simulink model "BrowarModel"  (R2024a)
settings: Solver=ode5  StartTime=0.0  StopTime=inf  FixedStep=0.1  RelTol=1e-3
undefined symbols (not defined in the file or in its folder): localhost, Matrikon, OI
libraries: opclib x24
(part 8 of 9)

== system BrowarModel/Kadz filtracji/Kadz filtracji/Zbiornik gorny/Silnik elektryczny ==
  note: Silnik elektryczny
  note: Uszkodzenie silnika
  Zalaczenie : Inport
  Zadane obroty : Inport  Port=2
  Obciazenie zew : Inport  Port=3
  Uszkodzenie : Inport  Port=4
  Abs : Abs  SaturateOnIntegerOverflow=off
  Add : Sum
  Add1 : Sum  Inputs=+-
  Const : Constant
  Gain : Gain
  "Hz -> obr/min" : Gain  Gain=60/2
  Inercja mechaniczna : TransferFcn  Denominator=[1 1]
  Poslizg : DotProduct  OutDataTypeStr=Inherit: Inherit via internal rule
  Poslizg jalowy : Constant  Value=0.04
  Poslizg od obciazenia : Gain  Gain=0.05
  Prad jalowy : Gain  Gain=0.5
  Prad nominalny (10A) : Constant  Value=10
  Relay : Relay  OnOutputValue=0  OffOutputValue=1
  Saturation [0,1] : Saturate  UpperLimit=1  LowerLimit=0
  "Saturation [0,1] " : Saturate  UpperLimit=1  LowerLimit=0
  Stan : Subsystem
  Sterowanie : Subsystem
  Sterownik : Subsystem
  Sum : Sum  Inputs=|+-
  Sum1 : Sum  Inputs=|++
  Sum2 : Sum  Inputs=|+-
  Sum3 : Sum  Inputs=|++
  Wplyw uszkodzenia : DotProduct  OutDataTypeStr=Inherit: Inherit via internal rule
  Wplyw obciazenia : DotProduct  OutDataTypeStr=Inherit: Inherit via internal rule
  Wplyw obrotow : DotProduct  OutDataTypeStr=Inherit: Inherit via internal rule
  Zaklocenia : Subsystem
  Zalaczony : DotProduct  OutDataTypeStr=Inherit: Inherit via internal rule
  "obr/min -> FS  " : Gain  Gain=1/1500
  "obr/min -> Hz" : Gain  Gain=1/60*2
  Obroty : Outport
  Prad : Outport  Port=2
  Idle : Outport  Port=3
  Running : Outport  Port=4
  Alarm : Outport  Port=5
  wires:
  Inercja mechaniczna/1 -> Obroty/1, Poslizg/1, Add1/2, "obr/min -> Hz"/1
  Sum/1 -> Inercja mechaniczna/1
  "Hz -> obr/min"/1 -> Sum2/1, Zaklocenia/1(In)  "[obr/min]"
  Poslizg/1 -> Sum/2
  Sum3/1 -> Poslizg/2
  Poslizg od obciazenia/1 -> Sum3/1
  Obciazenie zew/1 -> Saturation [0,1]/1  "FS"
  Poslizg jalowy/1 -> Sum3/2
  Prad nominalny (10A)/1 -> Prad jalowy/1  "A"
  Prad jalowy/1 -> Sum1/2, Wplyw obciazenia/2
  Wplyw obciazenia/1 -> Sum1/1
  Abs/1 -> Wplyw obciazenia/1  "FS"
  Const/1 -> Wplyw obrotow/1
  "obr/min -> Hz"/1 -> Sterownik/1(PV)
  Saturation [0,1]/1 -> Add/2
  Add/1 -> Poslizg od obciazenia/1, Abs/1  "FS"
  Add1/1 -> "obr/min -> FS  "/1
  "obr/min -> FS  "/1 -> Gain/1
  "Saturation [0,1] "/1 -> Add/1
  Zalaczenie/1 -> Sterowanie/2(Zalaczenie), Stan/1(Zalaczony)
  Sterowanie/1(Sterowanie) -> Sterownik/2(SP)
  Gain/1 -> "Saturation [0,1] "/1
  Uszkodzenie/1 -> Relay/1
  Sterownik/1(CV) -> Wplyw uszkodzenia/1
  Relay/1 -> Wplyw uszkodzenia/2, Stan/2(Zdatny)
  Wplyw uszkodzenia/1 -> "Hz -> obr/min"/1
  Wplyw obrotow/1 -> Prad/1  "A"
  Sum1/1 -> Zalaczony/1  "A"
  Zalaczony/1 -> Wplyw obrotow/2
  Zadane obroty/1 -> Sterowanie/1(Zadane obroty)
  Stan/1(Idle) -> Idle/1
  Stan/2(Running) -> Running/1, Zalaczony/2
  Stan/3(Alarm) -> Alarm/1
  Sum2/1 -> Add1/1, Sum/1
  Zaklocenia/1(Out) -> Sum2/2

== system BrowarModel/Kadz warzelna/Kadz warzelna/Model akumulacji ciepla w zbiorniku z ciecza/Cieplo strumienia cieczy doplywajacej ==
  Temperatura strumienia cieczy : Inport
  Strumien cieczy : Inport  Port=2
  "  Dot " : DotProduct  OutDataTypeStr=Inherit: Inherit via internal rule
  Cieplo wlasciwe : Constant  Value=4189.9
  Dot : DotProduct  OutDataTypeStr=Inherit: Inherit via internal rule
  Gestosc cieczy : Gain  Gain=1000
  Sum9 : Sum  Inputs=|++
  "Zamiana C->K " : Constant  Value=273.6
  Strumien ciepla : Outport
  wires:
  Cieplo wlasciwe/1 -> Dot/1  "J/(kg*K)"
  Sum9/1 -> Dot/2  "dec K"
  "Zamiana C->K "/1 -> Sum9/2
  Dot/1 -> "  Dot "/1
  Gestosc cieczy/1 -> "  Dot "/2  "kg/s"
  Temperatura strumienia cieczy/1 -> Sum9/1
  "  Dot "/1 -> Strumien ciepla/1  "J/s"
  Strumien cieczy/1 -> Gestosc cieczy/1

== system BrowarModel/Kadz warzelna/Kadz warzelna/Model akumulacji ciepla w zbiorniku z ciecza/Cieplo strumienia cieczy odplywajacej ==
  Temperatura strumienia cieczy : Inport
  Strumien cieczy : Inport  Port=2
  " Dot " : DotProduct  OutDataTypeStr=Inherit: Inherit via internal rule
  Cieplo wlasciwe : Constant  Value=4189.9
  "Dot " : DotProduct  OutDataTypeStr=Inherit: Inherit via internal rule
  Gestosc : Gain  Gain=1000
  Strumien ciepla : Outport
  wires:
  "Dot "/1 -> " Dot "/2
  Cieplo wlasciwe/1 -> "Dot "/2  "J/(kg*K)"
  Temperatura strumienia cieczy/1 -> " Dot "/1  "decK"
  Strumien cieczy/1 -> Gestosc/1  "m3/s"
  " Dot "/1 -> Strumien ciepla/1  "J/s"
  Gestosc/1 -> "Dot "/1  "kg/s"

== system BrowarModel/Kadz warzelna/Kadz warzelna/Model jakosci warzenia/Gotowanie  ==
  Srednia temperatura : Inport
  Jakosc mieszaniny : Inport  Port=2
  Objetosc mieszaniny : Inport  Port=3
  Odplyw : Inport  Port=4
  Booster : Product  RndMeth=Zero
  Booster block : Subsystem
  Display : Display
  Display1 : Display
  Divide : Product  Inputs=*/
  Dynamika rozkladu : Gain  Gain=1/1000
  Ilosc : Integrator  LimitOutput=on  UpperSaturationLimit=48  LowerSaturationLimit=0
  Nasycenie : DotProduct  OutDataTypeStr=Inherit: Inherit via internal rule
  "Odplyw " : DotProduct  OutDataTypeStr=Inherit: Inherit via internal rule
  Relational Operator1 : RelationalOperator  Operator=>  InputSameDT=off
  Sum8 : Sum  Inputs=|+-
  Sum9 : Sum  Inputs=|+-
  Szybkosc reakcji : DotProduct  OutDataTypeStr=Inherit: Inherit via internal rule
  Warunki rozkladu : DotProduct  OutDataTypeStr=Inherit: Inherit via internal rule
  Wplyw temperatury : Lookup  InputValues=[0, 80, 90, 95, 100]  Table=[0, 0, 0.9, 1, 1]  SaturateOnIntegerOverflow=off
  Jakosc : Outport
  wires:
  Wplyw temperatury/1 -> Warunki rozkladu/2, Display/1
  Warunki rozkladu/1 -> Dynamika rozkladu/1
  Ilosc/1 -> Sum8/2, Divide/1
  Divide/1 -> "Odplyw "/2, Relational Operator1/2, Jakosc/1, Display1/1
  Relational Operator1/1 -> Nasycenie/1
  Sum8/1 -> Szybkosc reakcji/2
  Sum9/1 -> Ilosc/1
  Nasycenie/1 -> Sum9/1
  "Odplyw "/1 -> Sum9/2
  Srednia temperatura/1 -> Wplyw temperatury/1
  Objetosc mieszaniny/1 -> Divide/2, Sum8/1
  Odplyw/1 -> "Odplyw "/1
  Jakosc mieszaniny/1 -> Warunki rozkladu/1, Relational Operator1/1
  Booster block/1(Out) -> Booster/1
  Szybkosc reakcji/1 -> Nasycenie/2
  Dynamika rozkladu/1 -> Booster/2
  Booster/1 -> Szybkosc reakcji/1

== system BrowarModel/Kadz warzelna/Kadz warzelna/Model ogrzewacza/Booster  ==
  In1 : Inport
  In2 : Inport  Port=2
  Switch : Switch  Threshold=0.5  SaturateOnIntegerOverflow=off  InputSameDT=off
  Out : Outport
  wires:
  [TrybSym] -> Switch/2
  In1/1 -> Switch/1
  Switch/1 -> Out/1
  In2/1 -> Switch/3

== system BrowarModel/Kadz warzelna/Kadz warzelna/Model ogrzewacza/Booster block ==
  Fast : Constant  Value=2
  Normal : Constant
  Switch : Switch  Threshold=0.5  SaturateOnIntegerOverflow=off  InputSameDT=off
  Out : Outport
  wires:
  [TrybSym] -> Switch/2
  Fast/1 -> Switch/1
  Normal/1 -> Switch/3
  Switch/1 -> Out/1

== system BrowarModel/Kadz warzelna/Kadz warzelna/Model ogrzewacza/Zaklocenia ==
  note: Zaklocenia procesowe
  In : Inport
  Product3 : Product  InputSameDT=on  RndMeth=Zero  SaturateOnIntegerOverflow=on  OutDataTypeStr=Inherit: Same as first input
  Product4 : Product  InputSameDT=on  RndMeth=Zero  SaturateOnIntegerOverflow=on  OutDataTypeStr=Inherit: Same as first input
  Random Number : RandomNumber  Seed=4365624  SampleTime=0.1
  Transfer Fcn1 : TransferFcn  Denominator=[10 1]
  Transfer Fcn2 : TransferFcn  Denominator=[10 1]
  Transfer Fcn3 : TransferFcn  Denominator=[10 1]
  Out : Outport
  wires:
  [ZaklProc] -> Product3/2
  Random Number/1 -> Product3/1
  Product3/1 -> Transfer Fcn1/1
  Transfer Fcn1/1 -> Transfer Fcn2/1
  In/1 -> Product4/1
  Product4/1 -> Out/1
  Transfer Fcn2/1 -> Transfer Fcn3/1
  Transfer Fcn3/1 -> Product4/2

== system BrowarModel/Kadz warzelna/Kadz warzelna/Model rozkladu temperatur/Model rozkladu temperatur ==
  Poziom : Inport
  Temperatura otoczenia : Inport  Port=2
  Srednia temperatura : Inport  Port=3
  "  1/2  " : Gain  Gain=0.5
  "  1/2  1" : Gain  Gain=2
  " Dot  1" : DotProduct  OutDataTypeStr=Inherit: Inherit via internal rule
  "1/2  " : Gain  Gain=0.5
  Max gradient : Gain  Gain=0.9
  MinMax : MinMax
  Mux : Mux  Inputs=2
  Poziom FS : Gain  Gain=1/3
  Sat doplyw Sat FS1 : Saturate  UpperLimit=1  LowerLimit=0
  Saturation : Saturate  UpperLimit=100  LowerLimit=0
  Saturation1 : Saturate  UpperLimit=100  LowerLimit=0
  Saturation2 : Saturate  UpperLimit=100  LowerLimit=0
  Sum1 : Sum  Inputs=|++
  Sum2 : Sum  Inputs=|-+
  Sum3 : Sum  Inputs=|+-
  Sum4 : Sum  Inputs=|-+
  Sum5 : Sum  Inputs=|++
  Sum7 : Sum  Inputs=|-+
  Sum8 : Sum  Inputs=|++
  Transfer Fcn : TransferFcn  Denominator=[10 1]
  Temperatura przy powierzchni : Outport
  Temperatura przy dnie : Outport  Port=2
  Gradient temperatury : Outport  Port=3
  wires:
  Srednia temperatura/1 -> Sum8/2, Sum4/2, Sum1/2, Sum2/2, Sum3/2, Sum5/2, Sum7/2
  Transfer Fcn/1 -> Sat doplyw Sat FS1/1
  Max gradient/1 -> Transfer Fcn/1
  Poziom FS/1 -> Max gradient/1
  Sat doplyw Sat FS1/1 -> " Dot  1"/1
  Sum4/1 -> " Dot  1"/2
  " Dot  1"/1 -> "1/2  "/1, "  1/2  "/1
  "1/2  "/1 -> Sum1/1
  "  1/2  "/1 -> Sum2/1
  Sum2/1 -> Saturation/1
  Sum1/1 -> Saturation1/1
  Saturation1/1 -> Sum3/1
  Saturation/1 -> Sum5/1
  Sum5/1 -> Mux/1
  Sum3/1 -> Mux/2
  Mux/1 -> MinMax/1
  MinMax/1 -> Saturation2/1
  Saturation2/1 -> Sum8/1, Sum7/1, "  1/2  1"/1
  Poziom/1 -> Poziom FS/1
  Temperatura otoczenia/1 -> Sum4/1
  Sum7/1 -> Temperatura przy powierzchni/1
  "  1/2  1"/1 -> Gradient temperatury/1
  Sum8/1 -> Temperatura przy dnie/1

== system BrowarModel/Kadz warzelna/Kadz warzelna/Odplyw z kadzi/Silnik elektryczny ==
  note: Silnik elektryczny
  note: Uszkodzenie silnika
  Zalaczenie : Inport
  Zadane obroty : Inport  Port=2
  Obciazenie zew : Inport  Port=3
  Uszkodzenie : Inport  Port=4
  Abs : Abs  SaturateOnIntegerOverflow=off
  Add : Sum
  Add1 : Sum  Inputs=+-
  Const : Constant
  Gain : Gain
  "Hz -> obr/min" : Gain  Gain=60/2
  Inercja mechaniczna : TransferFcn  Denominator=[1 1]
  Poslizg : DotProduct  OutDataTypeStr=Inherit: Inherit via internal rule
  Poslizg jalowy : Constant  Value=0.04
  Poslizg od obciazenia : Gain  Gain=0.05
  Prad jalowy : Gain  Gain=0.5
  Prad nominalny (10A) : Constant  Value=10
  Relay : Relay  OnOutputValue=0  OffOutputValue=1
  Saturation [0,1] : Saturate  UpperLimit=1  LowerLimit=0
  "Saturation [0,1] " : Saturate  UpperLimit=1  LowerLimit=0
  Stan : Subsystem
  Sterowanie : Subsystem
  Sterownik : Subsystem
  Sum : Sum  Inputs=|+-
  Sum1 : Sum  Inputs=|++
  Sum2 : Sum  Inputs=|+-
  Sum3 : Sum  Inputs=|++
  Wplyw uszkodzenia : DotProduct  OutDataTypeStr=Inherit: Inherit via internal rule
  Wplyw obciazenia : DotProduct  OutDataTypeStr=Inherit: Inherit via internal rule
  Wplyw obrotow : DotProduct  OutDataTypeStr=Inherit: Inherit via internal rule
  Zaklocenia : Subsystem
  Zalaczony : DotProduct  OutDataTypeStr=Inherit: Inherit via internal rule
  "obr/min -> FS  " : Gain  Gain=1/1500
  "obr/min -> Hz" : Gain  Gain=1/60*2
  Obroty : Outport
  Prad : Outport  Port=2
  Idle : Outport  Port=3
  Running : Outport  Port=4
  Alarm : Outport  Port=5
  wires:
  Inercja mechaniczna/1 -> Obroty/1, Poslizg/1, Add1/2, "obr/min -> Hz"/1
  Sum/1 -> Inercja mechaniczna/1
  "Hz -> obr/min"/1 -> Sum2/1, Zaklocenia/1(In)  "[obr/min]"
  Poslizg/1 -> Sum/2
  Sum3/1 -> Poslizg/2
  Poslizg od obciazenia/1 -> Sum3/1
  Obciazenie zew/1 -> Saturation [0,1]/1  "FS"
  Poslizg jalowy/1 -> Sum3/2
  Prad nominalny (10A)/1 -> Prad jalowy/1  "A"
  Prad jalowy/1 -> Sum1/2, Wplyw obciazenia/2
  Wplyw obciazenia/1 -> Sum1/1
  Abs/1 -> Wplyw obciazenia/1  "FS"
  Const/1 -> Wplyw obrotow/1
  "obr/min -> Hz"/1 -> Sterownik/1(PV)
  Saturation [0,1]/1 -> Add/2
  Add/1 -> Poslizg od obciazenia/1, Abs/1  "FS"
  Add1/1 -> "obr/min -> FS  "/1
  "obr/min -> FS  "/1 -> Gain/1
  "Saturation [0,1] "/1 -> Add/1
  Zalaczenie/1 -> Sterowanie/2(Zalaczenie), Stan/1(Zalaczony)
  Sterowanie/1(Sterowanie) -> Sterownik/2(SP)
  Gain/1 -> "Saturation [0,1] "/1
  Uszkodzenie/1 -> Relay/1
  Sterownik/1(CV) -> Wplyw uszkodzenia/1
  Relay/1 -> Wplyw uszkodzenia/2, Stan/2(Zdatny)
  Wplyw uszkodzenia/1 -> "Hz -> obr/min"/1
  Wplyw obrotow/1 -> Prad/1  "A"
  Sum1/1 -> Zalaczony/1  "A"
  Zalaczony/1 -> Wplyw obrotow/2
  Zadane obroty/1 -> Sterowanie/1(Zadane obroty)
  Stan/1(Idle) -> Idle/1
  Stan/2(Running) -> Running/1, Zalaczony/2
  Stan/3(Alarm) -> Alarm/1
  Sum2/1 -> Add1/1, Sum/1
  Zaklocenia/1(Out) -> Sum2/2

== system BrowarModel/Kadz warzelna/Kadz warzelna/Odplyw z kadzi/Zawor dyskretny ==
  note: Model zaworu dyskretnego
  Sterowanie : Inport
  Cisnienie : Inport  Port=2
  Przeciek : Inport  Port=3
  Dlawienie : Inport  Port=4
  Const : Constant  Value=100
  GUIMon : Gain
  Gain : Gain  Gain=(0.15/sqrt(300))/100
  Gain1 : Gain  Gain=1/100
  Integer Delay : Delay  DelayLength=15
  Math Function : Math  Operator=sqrt  SignedPower=on
  Product : Product  RndMeth=Zero
  Product1 : Product  RndMeth=Zero
  Relay : Relay  OnOutputValue=100
  Sat (0-100) : Saturate  UpperLimit=100  LowerLimit=0
  Sat dlawienia (0-100) : Saturate  UpperLimit=100  LowerLimit=0
  Sat przecieku (0-100) : Saturate  UpperLimit=100  LowerLimit=0
  Sum3 : Sum  Inputs=|+-
  Sum4 : Sum  Inputs=|++
  Transfer Fcn : TransferFcn  Denominator=[0.2 1]
  Przeplyw : Outport
  wires:
  Const/1 -> Sum3/1
  Sat dlawienia (0-100)/1 -> Sum3/2
  Sum3/1 -> Gain1/1
  Sat (0-100)/1 -> Product/1
  Sum4/1 -> Sat (0-100)/1
  Relay/1 -> GUIMon/1
  Sat przecieku (0-100)/1 -> Sum4/2
  Sterowanie/1 -> Relay/1
  Product/1 -> Product1/2  "[0,1]"
  Przeciek/1 -> Sat przecieku (0-100)/1
  Dlawienie/1 -> Sat dlawienia (0-100)/1
  Product1/1 -> Transfer Fcn/1
  Gain/1 -> Integer Delay/1  "m3/s"
  Cisnienie/1 -> Math Function/1  "kPa"
  Math Function/1 -> Product1/1
  Transfer Fcn/1 -> Gain/1
  Integer Delay/1 -> Przeplyw/1
  GUIMon/1 -> Sum4/1
  Gain1/1 -> Product/2

== system BrowarModel/Kadz zacierna/Kadz zacierna/Kadz zacierna/Model akumulacji ciepla w zbiorniku z ciecza ==
  note: Model akumulacji ciepla w zbiorniku
  Objetosc cieczy w zbiorniku : Inport
  Przepelnienie : Inport  Port=2
  Strumien odplywu cieczy : Inport  Port=3
  Strumien doplywu wody : Inport  Port=4
  Strumien sruty : Inport  Port=5
  Temperatura strumien doplywu wody : Inport  Port=6
  Temperatura strumien doplywu sruty : Inport  Port=7
  Strumien cieplna dostepny : Inport  Port=8
  Strumien cieplo traconego : Inport  Port=9
  1/gestosc cieczy : Gain  Gain=1/1000
  Cieplo : Integrator  InitialCondition=1238534.44  LimitOutput=on  LowerSaturationLimit=0
  Cieplo parowania : Constant  Value=2257000
  Cieplo strumienia cieczy odplywajacej : Subsystem
  Cieplo strumienia doplywajacego : Subsystem
  "Cieplo wlasciwe " : Constant  Value=4189.9
  Divide : Product  Inputs=/*
  Divide1 : Product  Inputs=*/
  Divide2 : Product  Inputs=*/
  "Dot " : DotProduct  OutDataTypeStr=Inherit: Inherit via internal rule
  Dot 1 : DotProduct  OutDataTypeStr=Inherit: Inherit via internal rule
  Gestosc cieczy : Gain  Gain=1000
  Saturation : Saturate  UpperLimit=inf  LowerLimit=0
  Sum{1..2,4..5} (4 alike) : Sum  Inputs=|+-
  Sum10 : Sum  Inputs=|++
  Sum3 : Sum  Inputs=|-+
  Sum7 : Sum  Inputs=|++
  Switch : Switch  Threshold=0.5  SaturateOnIntegerOverflow=off  InputSameDT=off
  Switch1 : Switch  Threshold=-0.5  SaturateOnIntegerOverflow=off  InputSameDT=off
  Temperatura parowania : Constant  Value=100
  Zamiana C->K : Constant  Value=273.6
  Zero : Constant  Value=0
  Srumien cieczy odparowanej : Outport
  Srednia temperaturacie czy : Outport  Port=2
  wires:
  Strumien odplywu cieczy/1 -> Sum7/1  "m3/s"
  Sum7/1 -> Cieplo strumienia cieczy odplywajacej/2(Strumien cieczy)
  Gestosc cieczy/1 -> Divide/1, "Dot "/2  "kg"
  Objetosc cieczy w zbiorniku/1 -> Gestosc cieczy/1  "m3"
  Cieplo parowania/1 -> Divide2/2  "J/kg"
  Divide2/1 -> 1/gestosc cieczy/1  "kg/s"
  1/gestosc cieczy/1 -> Srumien cieczy odparowanej/1, Sum7/2  "m3/s"
  Sum2/1 -> Cieplo/1  "J/s"
  "Dot "/1 -> Sum2/2, Divide2/1  "J/s"
  Dot 1/1 -> "Dot "/1
  Saturation/1 -> Dot 1/1
  Sum4/1 -> Saturation/1
  Temperatura parowania/1 -> Sum4/2  "dec C"
  Sum10/1 -> Sum2/1  "J/s"
  Sum1/1 -> Sum10/1  "J/s"
  Strumien cieplo traconego/1 -> Sum1/2  "J/s"
  Sum3/1 -> Sum1/1  "J/s"
  Cieplo/1 -> Divide/2  "J"
  Divide/1 -> Divide1/1
  Divide1/1 -> Cieplo strumienia cieczy odplywajacej/1(Temperatura strumienia cieczy), Sum5/1  "dec K"
  Temperatura strumien doplywu wody/1 -> Cieplo strumienia doplywajacego/1(Temperatura strumienia wody)  "dec C"
  "Cieplo wlasciwe "/1 -> Dot 1/2, Divide1/2  "J/(kg*K)"
  Zamiana C->K/1 -> Sum5/2
  Strumien doplywu wody/1 -> Cieplo strumienia doplywajacego/2(Strumien wody)  "m3/s"
  Sum5/1 -> Sum4/1, Srednia temperaturacie czy/1
  Strumien cieplna dostepny/1 -> Sum10/2  "J/s"
  Strumien sruty/1 -> Cieplo strumienia doplywajacego/4(Strumien sruty)
  Temperatura strumien doplywu sruty/1 -> Cieplo strumienia doplywajacego/3(Temperatura strumienia sruty)
  Przepelnienie/1 -> Switch/2, Switch1/2
  Cieplo strumienia doplywajacego/1(Strumien ciepla) -> Switch/3  "J/s"
  Switch/1 -> Sum3/2
  Cieplo strumienia cieczy odplywajacej/1(Strumien ciepla) -> Switch/1, Switch1/1  "J/s"
  Switch1/1 -> Sum3/1
  Zero/1 -> Switch1/3

== system BrowarModel/Kadz zacierna/Kadz zacierna/Kadz zacierna/Model jakosci zacieru ==
  note: Model jakosci zacieru
  Srednia temperatura : Inport
  Odplyw : Inport  Port=2
  Doplyw wody : Inport  Port=3
  Doplyw srutu : Inport  Port=4
  Obroty mieszadla : Inport  Port=5
  Constant : Constant  Value=48
  Display{,1..3} (4 alike) : Display
  Divide : Product  Inputs=*/
  Divide1 : Product  Inputs=/*
  Jakosc mieszaniny : Lookup  InputValues=[0, 0.5 0.75, 1]  Table=[0, 0.1 1, 0]  SaturateOnIntegerOverflow=off
  Objetosc srutu : Integrator  InitialCondition=0.001  LimitOutput=on  UpperSaturationLimit=48  LowerSaturationLimit=0.001
  Objetosc wody : Integrator  InitialCondition=0.001  LimitOutput=on  UpperSaturationLimit=48  LowerSaturationLimit=0.001
  Obroty skalowanie : Gain  Gain=1/2
  Odplyw srutu : DotProduct  OutDataTypeStr=Inherit: Inherit via internal rule
  Odplyw wody : DotProduct  OutDataTypeStr=Inherit: Inherit via internal rule
  Przepelnienie - srut : DotProduct  OutDataTypeStr=Inherit: Inherit via internal rule
  Przepelnienie - woda : DotProduct  OutDataTypeStr=Inherit: Inherit via internal rule
  "Przerwa bialkowa " : Subsystem
  Przerwa dekstrynujaca : Subsystem
  Przerwa maltozowa : Subsystem
  Relational Operator : RelationalOperator  Operator=<  InputSameDT=off
  Sat doplyw Sat FS : Saturate  UpperLimit=1  LowerLimit=0
  Saturation : Saturate  UpperLimit=inf  LowerLimit=0
  Sum5 : Sum  Inputs=-+
  Sum6 : Sum  Inputs=+-
  Sum7 : Sum
  Jakosc : Outport
  wires:
  Sum6/1 -> Objetosc srutu/1
  Odplyw srutu/1 -> Sum6/2
  Objetosc wody/1 -> Sum7/1, Divide/1
  Objetosc srutu/1 -> Sum7/2, Divide1/2
  Sum7/1 -> Divide1/1, Divide/2, Relational Operator/1, "Przerwa bialkowa "/3(Objetosc mieszaniny), Przerwa maltozowa/4(Objetosc mieszaniny), Przerwa dekstrynujaca/4(Objetosc mieszaniny)  "m3"
  Odplyw wody/1 -> Sum5/1
  Divide/1 -> Odplyw wody/1, Jakosc mieszaniny/1
  Divide1/1 -> Odplyw srutu/2
  Sum5/1 -> Objetosc wody/1
  Przepelnienie - woda/1 -> Sum5/2
  Przepelnienie - srut/1 -> Sum6/1
  Relational Operator/1 -> Przepelnienie - woda/2, Przepelnienie - srut/1
  Constant/1 -> Relational Operator/2
  "Przerwa bialkowa "/1(Skrobia rozpuszczona) -> Przerwa maltozowa/1(Skrobia rozpuszczona), Display1/1
  Przerwa maltozowa/1(Dekstryny) -> Przerwa dekstrynujaca/1(Dekstryny), Display2/1
  Srednia temperatura/1 -> "Przerwa bialkowa "/1(Srednia temperatura), Przerwa maltozowa/2(Srednia temperatura), Przerwa dekstrynujaca/2(Srednia temperatura)  "decC"
  Odplyw/1 -> Odplyw wody/2, Odplyw srutu/1, Przerwa dekstrynujaca/5(Odplyw), "Przerwa bialkowa "/4(Odplyw), Przerwa maltozowa/5(Odplyw)  "m3/s"
  Doplyw wody/1 -> Przepelnienie - woda/1  "m3/s"
  Doplyw srutu/1 -> Przepelnienie - srut/2  "m3/s"
  Przerwa dekstrynujaca/1(Maltoza) -> Saturation/1, Display3/1
  Jakosc mieszaniny/1 -> "Przerwa bialkowa "/2(Jakosc mieszaniny), Przerwa maltozowa/3(Jakosc mieszaniny), Przerwa dekstrynujaca/3(Jakosc mieszaniny), Display/1  "[0,1]"
  Saturation/1 -> Jakosc/1
  Obroty skalowanie/1 -> Sat doplyw Sat FS/1  "FS"
  Obroty mieszadla/1 -> Obroty skalowanie/1  "obr/min"
  Sat doplyw Sat FS/1 -> "Przerwa bialkowa "/5(Obroty mieszadla), Przerwa maltozowa/6(Obroty mieszadla), Przerwa dekstrynujaca/6(Obroty mieszadla)

== system BrowarModel/Kadz zacierna/Kadz zacierna/Kadz zacierna/Model rozkladu temperatur ==
  note: Model rozkladu temperatury
  Poziom : Inport
  Srednia temperatura : Inport  Port=2
  Obroty mieszadla : Inport  Port=3
  " Dot 1" : DotProduct  OutDataTypeStr=Inherit: Inherit via internal rule
  " Dot 2" : DotProduct  OutDataTypeStr=Inherit: Inherit via internal rule
  " Dot 3" : DotProduct  OutDataTypeStr=Inherit: Inherit via internal rule
  Divide2 : Product  Inputs=/*
  Divide3 : Product  Inputs=/*
  Divide4 : Product  Inputs=/*
  Gradient temperatury : Subsystem
  Pozycja sensor dolny : Constant  Value=0.4
  Pozycja sensor gorny : Constant  Value=1.2
  Pozycja sensor srodkowy : Constant  Value=0.8
  Sensor dolny niezanuzony : RelationalOperator  Operator=<  InputSameDT=off
  Sensor gorny niezanuzony : RelationalOperator  Operator=<  InputSameDT=off
  Sensor srodkowy niezanuzony : RelationalOperator  Operator=<  InputSameDT=off
  Sum13 : Sum  Inputs=|+-
  Sum14 : Sum  Inputs=|+-
  Sum15 : Sum  Inputs=|+-
  Switch : Switch  Threshold=0.5  SaturateOnIntegerOverflow=off  InputSameDT=off
  Switch1 : Switch  Threshold=0.5  SaturateOnIntegerOverflow=off  InputSameDT=off
  Switch2 : Switch  Threshold=0.5  SaturateOnIntegerOverflow=off  InputSameDT=off
  "Temperatura pokojowa (deg C) " : Constant  Value=22
  Temperatura lustra zbiornika : Outport
  Sensor temperatury gorny : Outport  Port=2
  Sensor temperatury srodkowy : Outport  Port=3
  Sensor temperatury dolny : Outport  Port=4
  Temperatura przy dnie zbiornika : Outport  Port=5
  wires:
  Obroty mieszadla/1 -> Gradient temperatury/4(Obroty mieszadla)  "obr/min"
  Srednia temperatura/1 -> Gradient temperatury/3(Srednia temperatura)  "decC"
  Gradient temperatury/3(Gradient temperatury) -> " Dot 3"/1, " Dot 2"/1, " Dot 1"/1
  "Temperatura pokojowa (deg C) "/1 -> Gradient temperatury/2(Temperatura otoczenia), Switch/1, Switch1/1, Switch2/1
  Pozycja sensor gorny/1 -> Sensor gorny niezanuzony/2, Divide4/2
  Pozycja sensor srodkowy/1 -> Sensor srodkowy niezanuzony/2, Divide3/2
  Pozycja sensor dolny/1 -> Sensor dolny niezanuzony/2, Divide2/2
  Sensor gorny niezanuzony/1 -> Switch/2
  Sensor srodkowy niezanuzony/1 -> Switch1/2
  Sensor dolny niezanuzony/1 -> Switch2/2
  Switch1/1 -> Sensor temperatury srodkowy/1
  Sum13/1 -> Switch/3
  Sum14/1 -> Switch1/3
  Sum15/1 -> Switch2/3
  Gradient temperatury/2(Temperatura przy dnie) -> Temperatura przy dnie zbiornika/1, Sum13/1, Sum14/1, Sum15/1
  Divide4/1 -> " Dot 1"/2
  " Dot 1"/1 -> Sum13/2
  " Dot 2"/1 -> Sum14/2
  Divide3/1 -> " Dot 2"/2
  Divide2/1 -> " Dot 3"/2
  " Dot 3"/1 -> Sum15/2
  Switch/1 -> Sensor temperatury gorny/1
  Switch2/1 -> Sensor temperatury dolny/1
  Poziom/1 -> Gradient temperatury/1(Poziom), Sensor gorny niezanuzony/1, Sensor srodkowy niezanuzony/1, Sensor dolny niezanuzony/1, Divide2/1, Divide3/1, Divide4/1  "m"
  Gradient temperatury/1(Temperatura przy powierzchni) -> Temperatura lustra zbiornika/1

== system BrowarModel/Kadz zacierna/Kadz zacierna/Kadz zacierna/Model utratu ciepla ==
  note: Model utraty ciepla
  Poziom : Inport
  Pole podstawy zbiornika : Inport  Port=2
  Srednia temperatura : Inport  Port=3
  Temperatura lustra : Inport  Port=4
  Cieplo tracone przez pow. gorna : DotProduct  OutDataTypeStr=Inherit: Inherit via internal rule
  Cieplo tracone przez scianki : DotProduct  OutDataTypeStr=Inherit: Inherit via internal rule
  Pow ->obwod : Fcn  Expr=2*3.14*sqrt(u(1)/3.14)
  Pow styku scian bocznych : DotProduct  OutDataTypeStr=Inherit: Inherit via internal rule
  Saturation : Saturate  UpperLimit=inf  LowerLimit=0
  Sum11 : Sum  Inputs=|-+
  Sum12 : Sum  Inputs=|-+
  Sum2 : Sum
  "Temperatura pokojowa (deg C)  " : Constant  Value=22
  Wspolczynnik przenikania ciepla : Gain  Gain=950
  Wspolczynnik przenikania ciepla scian : Gain  Gain=450
  Strumien ciepla : Outport
  wires:
  Saturation/1 -> Strumien ciepla/1  "J/s"
  Wspolczynnik przenikania ciepla/1 -> Cieplo tracone przez pow. gorna/2
  Sum12/1 -> Cieplo tracone przez pow. gorna/1
  Pow ->obwod/1 -> Pow styku scian bocznych/2
  Pow styku scian bocznych/1 -> Wspolczynnik przenikania ciepla scian/1  "m2"
  Wspolczynnik przenikania ciepla scian/1 -> Cieplo tracone przez scianki/1
  Cieplo tracone przez scianki/1 -> Sum2/1
  Cieplo tracone przez pow. gorna/1 -> Sum2/2
  "Temperatura pokojowa (deg C)  "/1 -> Sum11/1, Sum12/1
  Sum11/1 -> Cieplo tracone przez scianki/2
  Poziom/1 -> Pow styku scian bocznych/1
  Pole podstawy zbiornika/1 -> Pow ->obwod/1, Wspolczynnik przenikania ciepla/1
  Srednia temperatura/1 -> Sum11/2  "dec C"
  Sum2/1 -> Saturation/1
  Temperatura lustra/1 -> Sum12/2  "dec C"

== system BrowarModel/Kadz zacierna/Kadz zacierna/Kadz zacierna/Poziom zbiornika ==
  note: Poziom zbiornika
  Objetosc : Inport
  Powierzchnia dna : Inport  Port=2
  1/powierzchnia : Product  Inputs=*/
  Pozycja sensora max (2.8 m) : Constant  Value=1.3
  Pozycja sensora min (0.2 m) : Constant  Value=.15
  Sensor max : RelationalOperator  InputSameDT=off
  Sensor min : RelationalOperator  InputSameDT=off
  Poziom  wysoki : Outport
  Poziom niski : Outport  Port=2
  Poziom : Outport  Port=3
  wires:
  1/powierzchnia/1 -> Sensor min/1, Sensor max/1, Poziom/1  "m"
  Pozycja sensora max (2.8 m)/1 -> Sensor max/2
  Pozycja sensora min (0.2 m)/1 -> Sensor min/2
  Sensor max/1 -> Poziom  wysoki/1
  Sensor min/1 -> Poziom niski/1
  Powierzchnia dna/1 -> 1/powierzchnia/2  "m2"
  Objetosc/1 -> 1/powierzchnia/1  "m3"

== system BrowarModel/Kadz zacierna/Kadz zacierna/Model ogrzewacza/Booster  ==
  In1 : Inport
  In2 : Inport  Port=2
  Switch : Switch  Threshold=0.5  SaturateOnIntegerOverflow=off  InputSameDT=off
  Out : Outport
  wires:
  [TrybSym] -> Switch/2
  In1/1 -> Switch/1
  Switch/1 -> Out/1
  In2/1 -> Switch/3

== system BrowarModel/Kadz zacierna/Kadz zacierna/Model ogrzewacza/Booster block ==
  Fast : Constant  Value=2
  Normal : Constant
  Switch : Switch  Threshold=0.5  SaturateOnIntegerOverflow=off  InputSameDT=off
  Out : Outport
  wires:
  [TrybSym] -> Switch/2
  Fast/1 -> Switch/1
  Normal/1 -> Switch/3
  Switch/1 -> Out/1

== system BrowarModel/Kadz zacierna/Kadz zacierna/Model ogrzewacza/Zaklocenia ==
  note: Zaklocenia procesowe
  In : Inport
  Product3 : Product  InputSameDT=on  RndMeth=Zero  SaturateOnIntegerOverflow=on  OutDataTypeStr=Inherit: Same as first input
  Product4 : Product  InputSameDT=on  RndMeth=Zero  SaturateOnIntegerOverflow=on  OutDataTypeStr=Inherit: Same as first input
  Random Number : RandomNumber  Seed=4365624  SampleTime=0.1
  Transfer Fcn1 : TransferFcn  Denominator=[10 1]
  Transfer Fcn2 : TransferFcn  Denominator=[10 1]
  Transfer Fcn3 : TransferFcn  Denominator=[10 1]
  Out : Outport
  wires:
  [ZaklProc] -> Product3/2
  Random Number/1 -> Product3/1
  Product3/1 -> Transfer Fcn1/1
  Transfer Fcn1/1 -> Transfer Fcn2/1
  In/1 -> Product4/1
  Product4/1 -> Out/1
  Transfer Fcn2/1 -> Transfer Fcn3/1
  Transfer Fcn3/1 -> Product4/2

== system BrowarModel/Kadz zacierna/Kadz zacierna/Silnik elektryczny/Stan ==
  Zalaczony : Inport
  Zdatny : Inport  Port=2
  Add : Sum  Inputs=+++
  Alarm1 : Logic  Operator=NOT  AllPortsSameDT=off
  Alarm2 : Gain  Gain=3
  Display : Display
  GUIMon : Gain
  Idle1 : Logic  AllPortsSameDT=off
  Idle2 : Logic  Operator=NOT  AllPortsSameDT=off
  Idle3 : Gain
  Running1 : Logic  AllPortsSameDT=off
  Running2 : Gain  Gain=2
  Idle : Outport
  Running : Outport  Port=2
  Alarm : Outport  Port=3
  wires:
  Running1/1 -> Running/1, Running2/1
  Idle1/1 -> Idle/1, Idle3/1
  Zalaczony/1 -> Running1/1, Idle2/1
  Zdatny/1 -> Alarm1/1, Running1/2, Idle1/2
  Alarm1/1 -> Alarm/1, Alarm2/1
  Idle2/1 -> Idle1/1
  Idle3/1 -> Add/1
  Running2/1 -> Add/2
  Alarm2/1 -> Add/3
  Add/1 -> GUIMon/1
  GUIMon/1 -> Display/1

== system BrowarModel/Kadz zacierna/Kadz zacierna/Silnik elektryczny/Sterowanie ==
  note: Sterowanie silnika elektrycznego
  Zadane obroty : Inport
  Zalaczenie : Inport  Port=2
  Hz : Gain  Gain=45/100
  Min sterowanie : Constant  Value=5
  Relay : Relay
  Saturation [0,100] : Saturate  UpperLimit=100  LowerLimit=0
  "Sterowanie " : DotProduct  OutDataTypeStr=Inherit: Inherit via internal rule
  Sum2 : Sum  Inputs=|++
  Sterowanie : Outport
  wires:
  Relay/1 -> "Sterowanie "/1  "{0,1}"
  Saturation [0,100]/1 -> Hz/1
  Hz/1 -> Sum2/1  "Hz"
  Min sterowanie/1 -> Sum2/2  "Hz"
  Sum2/1 -> "Sterowanie "/2
  Zalaczenie/1 -> Relay/1  "{0,1}"
  "Sterowanie "/1 -> Sterowanie/1  "Hz"
  Zadane obroty/1 -> Saturation [0,100]/1  "[0,100]"

== system BrowarModel/Kadz zacierna/Kadz zacierna/Silnik elektryczny/Sterownik ==
  PV : Inport
  SP : Inport  Port=2
  Integrator : Integrator  LimitOutput=on  UpperSaturationLimit=50  LowerSaturationLimit=0
  K : Gain
  Saturation [0,50] : Saturate  UpperLimit=50  LowerLimit=0
  Sum2 : Sum  Inputs=|+-
  Sum3 : Sum  Inputs=|++
  Ti : Gain
  CV : Outport
  wires:
  Sum2/1 -> K/1
  Integrator/1 -> Sum3/1
  K/1 -> Ti/1, Sum3/2
  Ti/1 -> Integrator/1
  PV/1 -> Sum2/2
  SP/1 -> Sum2/1
  Sum3/1 -> Saturation [0,50]/1
  Saturation [0,50]/1 -> CV/1

== system BrowarModel/Kadz zacierna/Kadz zacierna/Silnik elektryczny/Zaklocenia ==
  note: Zaklocenia procesowe
  In : Inport
  Product3 : Product  InputSameDT=on  RndMeth=Zero  SaturateOnIntegerOverflow=on  OutDataTypeStr=Inherit: Same as first input
  Product4 : Product  InputSameDT=on  RndMeth=Zero  SaturateOnIntegerOverflow=on  OutDataTypeStr=Inherit: Same as first input
  Random Number : RandomNumber  Variance=0.05  Seed=4365624  SampleTime=0.1
  Transfer Fcn1 : TransferFcn  Denominator=[1 1]
  Transfer Fcn2 : TransferFcn  Denominator=[1 1]
  Transfer Fcn3 : TransferFcn  Denominator=[1 1]
  Out : Outport
  wires:
  [ZaklProc] -> Product3/2
  Random Number/1 -> Product3/1
  Product3/1 -> Transfer Fcn1/1
  Transfer Fcn1/1 -> Transfer Fcn2/1
  In/1 -> Product4/1
  Product4/1 -> Out/1
  Transfer Fcn2/1 -> Transfer Fcn3/1
  Transfer Fcn3/1 -> Product4/2

== system BrowarModel/Kadz zacierna/Kadz zacierna/Zawor doplywu wody/Booster block ==
  Fast : Constant  Value=2
  Normal : Constant
  Switch : Switch  Threshold=0.5  SaturateOnIntegerOverflow=off  InputSameDT=off
  Out : Outport
  wires:
  [TrybSym] -> Switch/2
  Fast/1 -> Switch/1
  Normal/1 -> Switch/3
  Switch/1 -> Out/1

== system BrowarModel/Kadz zacierna/Kadz zacierna/Zawor doplywu wody/Zaklocenia ==
  note: Zaklocenia procesowe
  In : Inport
  Product3 : Product  InputSameDT=on  RndMeth=Zero  SaturateOnIntegerOverflow=on  OutDataTypeStr=Inherit: Same as first input
  Product4 : Product  InputSameDT=on  RndMeth=Zero  SaturateOnIntegerOverflow=on  OutDataTypeStr=Inherit: Same as first input
  Random Number : RandomNumber  Variance=0.01  Seed=4365624  SampleTime=0.1
  Transfer Fcn1 : TransferFcn  Denominator=[0.1 1]
  Out : Outport
  wires:
  [ZaklProc] -> Product3/2
  Random Number/1 -> Product3/1
  Product3/1 -> Transfer Fcn1/1
  Transfer Fcn1/1 -> Product4/2
  In/1 -> Product4/1
  Product4/1 -> Out/1

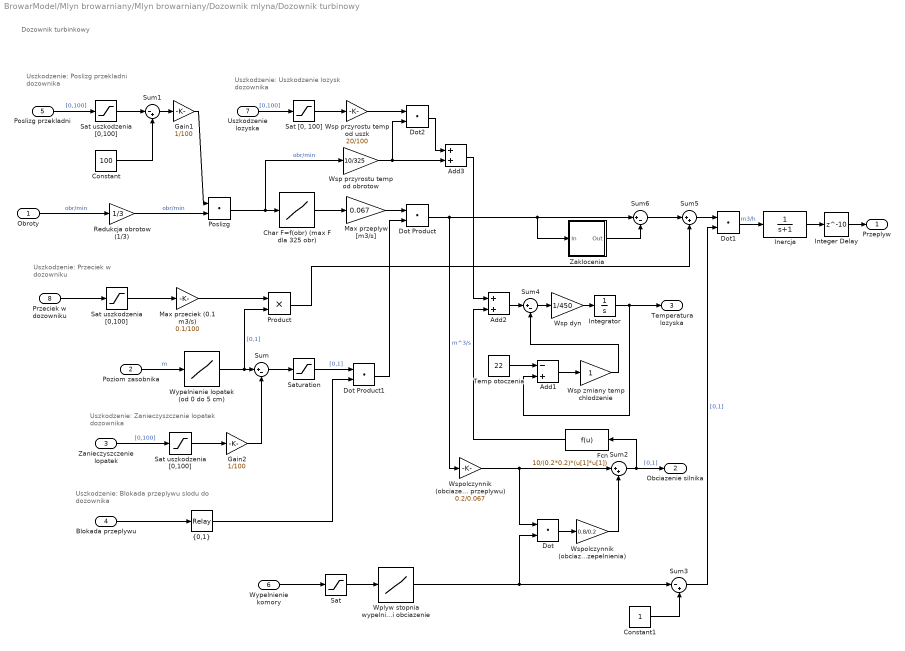
== system BrowarModel/Mlyn browarniany/Mlyn browarniany/Dozownik mlyna/Dozownik turbinowy ==
  note: Dozownik turbinkowy
  note: Uszkodzenie:
      | Poslizg przekladni dozownika
  note: Uszkodzenie:
      | Uszkodzenie lozysk dozownika
  note: Uszkodzenie:
      | Przeciek w dozowniku
  note: Uszkodzenie:
      | Zanieczyszczenie lopatek dozownika
  note: Uszkodzenie:
      | Blokada przeplywu slodu do dozownika
  Obroty : Inport
  Poziom zasobnika : Inport  Port=2
  Zanieczyszczenie lopatek : Inport  Port=3
  Blokada przeplywu : Inport  Port=4
  Poslizg przekladni : Inport  Port=5
  Wypelnienie komory : Inport  Port=6
  Uszkodzenie lozyska : Inport  Port=7
  Przeciek w dozowniku : Inport  Port=8
  Add1 : Sum  Inputs=-+
  Add2 : Sum
  Add3 : Sum
  Char F=f(obr) (max F dla 325 obr) : Lookup  InputValues="[0\t25\t50\t75\t100\t125\t150\t175\t200\t225\t250\t275\t300\t325\t350\t375\t400\t425\t450 475 500]"  Table="[0.0000\t0.1109\t0.2206\t0.3279\t0.4316\t0.5304\t0.6233\t0.7089\t0.7860\t0.8535\t0.9102\t0.9548\t0.9861\t1.0030\t1.0042\t0.9885\t0.9547\t0.9017\t0.8281\t0.7329\t0.6147]"  SaturateOnIntegerOverflow=off
  Constant : Constant  Value=100
  Constant1 : Constant
  Dot : DotProduct  OutDataTypeStr=Inherit: Inherit via internal rule
  Dot Product : DotProduct  OutDataTypeStr=Inherit: Inherit via internal rule
  Dot Product1 : DotProduct  OutDataTypeStr=Inherit: Inherit via internal rule
  Dot1 : DotProduct  OutDataTypeStr=Inherit: Inherit via internal rule
  Dot2 : DotProduct  OutDataTypeStr=Inherit: Inherit via internal rule
  Fcn : Fcn  Expr=10/(0.2*0.2)*(u[1]*u[1])
  Gain1 : Gain  Gain=1/100
  Gain2 : Gain  Gain=1/100
  Inercja : TransferFcn  Denominator=[1 1]
  Integer Delay : Delay  DelayLength=10
  Integrator : Integrator  InitialCondition=22  LimitOutput=on  LowerSaturationLimit=0
  Max przeciek (0.1 m3/s) : Gain  Gain=0.1/100
  Max przeplyw [m3/s] : Gain  Gain=0.067
  Poslizg : DotProduct  OutDataTypeStr=Inherit: Inherit via internal rule
  Product : Product  RndMeth=Zero
  Redukcja obrotow (1/3) : Gain  Gain=1/3
  Sat : Saturate  UpperLimit=1  LowerLimit=0
  "Sat [0, 100]" : Saturate  UpperLimit=100  LowerLimit=0
  Sat uszkodzenia [0,100] : Saturate  UpperLimit=100  LowerLimit=0
  "Sat uszkodzenia [0,100] " : Saturate  UpperLimit=100  LowerLimit=0
  "Sat uszkodzenia [0,100]  " : Saturate  UpperLimit=100  LowerLimit=0
  Saturation : Saturate  UpperLimit=1  LowerLimit=0
  Sum : Sum  Inputs=|+-
  Sum1 : Sum  Inputs=|-+
  Sum2 : Sum  Inputs=|++
  Sum3 : Sum  Inputs=|-+
  Sum4 : Sum  Inputs=|+-
  Sum5 : Sum  Inputs=|++
  Sum6 : Sum  Inputs=|+-
  Temp otoczenia : Constant  Value=22
  Wplyw stopnia wypelnienia na przeplyw i obciazenie : Lookup  InputValues=[0,0.9,1,2]  Table=[0,0,1,1]  SaturateOnIntegerOverflow=off
  Wsp dyn : Gain  Gain=1/450
  Wsp przyrostu temp od obrotow : Gain  Gain=10/325
  Wsp przyrostu temp od uszk : Gain  Gain=20/100
  Wsp zmiany temp chlodzenie : Gain
  Wspolczynnik (obciazenie od przepelnienia) : Gain  Gain=0.8/0.2
  Wspolczynnik (obciazenie od przeplywu) : Gain  Gain=0.2/0.067
  Wypelnienie lopatek (od 0 do 5 cm) : Lookup  InputValues=[-0.02,0,0.05,0.1]  Table=[0,0,1,1]  SaturateOnIntegerOverflow=off
  Zaklocenia : Subsystem
  "{0,1}" : Relay  OnOutputValue=0  OffOutputValue=1
  Przeplyw : Outport
  Obciazenie silnika : Outport  Port=2
  Temperatura lozyska : Outport  Port=3
  wires:
  Poziom zasobnika/1 -> Wypelnienie lopatek (od 0 do 5 cm)/1  "m"
  Obroty/1 -> Redukcja obrotow (1/3)/1  "obr/min"
  Char F=f(obr) (max F dla 325 obr)/1 -> Max przeplyw [m3/s]/1
  Max przeplyw [m3/s]/1 -> Dot Product/1
  Dot Product/1 -> Wspolczynnik (obciazenie od przeplywu)/1, Sum6/1, Zaklocenia/1(In)  "m^3/s"
  Wypelnienie lopatek (od 0 do 5 cm)/1 -> Sum/1, Product/2  "[0,1]"
  Sum/1 -> Saturation/1
  Zanieczyszczenie lopatek/1 -> "Sat uszkodzenia [0,100]  "/1  "[0,100]"
  "Sat uszkodzenia [0,100]  "/1 -> Gain2/1
  Redukcja obrotow (1/3)/1 -> Poslizg/2  "obr/min"
  Poslizg/1 -> Char F=f(obr) (max F dla 325 obr)/1, Wsp przyrostu temp od obrotow/1  "obr/min"
  Poslizg przekladni/1 -> Sat uszkodzenia [0,100]/1  "[0,100]"
  Sat uszkodzenia [0,100]/1 -> Sum1/1
  Sum1/1 -> Gain1/1
  Constant/1 -> Sum1/2
  Wypelnienie komory/1 -> Sat/1
  Sum2/1 -> Fcn/1, Obciazenie silnika/1  "[0,1]"
  Dot/1 -> Wspolczynnik (obciazenie od przepelnienia)/1
  Wplyw stopnia wypelnienia na przeplyw i obciazenie/1 -> Sum3/1, Dot/2
  Constant1/1 -> Sum3/2
  Sum3/1 -> Dot1/2  "[0,1]"
  Sum4/1 -> Wsp dyn/1
  Integrator/1 -> Add1/2, Temperatura lozyska/1
  Wspolczynnik (obciazenie od przeplywu)/1 -> Sum2/1, Dot/1
  Add1/1 -> Wsp zmiany temp chlodzenie/1
  Wsp zmiany temp chlodzenie/1 -> Sum4/2
  Uszkodzenie lozyska/1 -> "Sat [0, 100]"/1  "[0,100]"
  "Sat [0, 100]"/1 -> Wsp przyrostu temp od uszk/1
  Add2/1 -> Sum4/1
  Temp otoczenia/1 -> Add1/1
  Wsp przyrostu temp od obrotow/1 -> Add3/2, Dot2/2
  Wsp przyrostu temp od uszk/1 -> Dot2/1
  Dot2/1 -> Add3/1
  Add3/1 -> Add2/1
  Wsp dyn/1 -> Integrator/1
  Sat/1 -> Wplyw stopnia wypelnienia na przeplyw i obciazenie/1
  Saturation/1 -> Dot Product1/1  "[0,1]"
  Dot Product1/1 -> Dot Product/2
  Blokada przeplywu/1 -> "{0,1}"/1
  "{0,1}"/1 -> Dot Product1/2
  Dot1/1 -> Inercja/1  "m3/h"
  Inercja/1 -> Integer Delay/1
  Integer Delay/1 -> Przeplyw/1
  Fcn/1 -> Add2/2
  Gain1/1 -> Poslizg/1
  Sum5/1 -> Dot1/1
  Przeciek w dozowniku/1 -> "Sat uszkodzenia [0,100] "/1
  "Sat uszkodzenia [0,100] "/1 -> Max przeciek (0.1 m3/s)/1
  Max przeciek (0.1 m3/s)/1 -> Product/1
  Product/1 -> Sum5/2
  Gain2/1 -> Sum/2
  Wspolczynnik (obciazenie od przepelnienia)/1 -> Sum2/2
  Sum6/1 -> Sum5/1
  Zaklocenia/1(Out) -> Sum6/2

== system BrowarModel/Mlyn browarniany/Mlyn browarniany/Dozownik mlyna/Silnik elektryczny ==
  note: Silnik elektryczny
  note: Uszkodzenie silnika
  Zalaczenie : Inport
  Zadane obroty : Inport  Port=2
  Obciazenie zew : Inport  Port=3
  Uszkodzenie : Inport  Port=4
  Abs : Abs  SaturateOnIntegerOverflow=off
  Add : Sum
  Add1 : Sum  Inputs=+-
  Const : Constant
  Gain : Gain
  "Hz -> obr/min" : Gain  Gain=60/2
  Inercja mechaniczna : TransferFcn  Denominator=[1 1]
  Poslizg : DotProduct  OutDataTypeStr=Inherit: Inherit via internal rule
  Poslizg jalowy : Constant  Value=0.04
  Poslizg od obciazenia : Gain  Gain=0.05
  Prad jalowy : Gain  Gain=0.5
  Prad nominalny (10A) : Constant  Value=10
  Relay : Relay  OnOutputValue=0  OffOutputValue=1
  Saturation [0,1] : Saturate  UpperLimit=1  LowerLimit=0
  "Saturation [0,1] " : Saturate  UpperLimit=1  LowerLimit=0
  Stan : Subsystem
  Sterowanie : Subsystem
  Sterownik : Subsystem
  Sum : Sum  Inputs=|+-
  Sum1 : Sum  Inputs=|++
  Sum2 : Sum  Inputs=|+-
  Sum3 : Sum  Inputs=|++
  Wplyw uszkodzenia : DotProduct  OutDataTypeStr=Inherit: Inherit via internal rule
  Wplyw obciazenia : DotProduct  OutDataTypeStr=Inherit: Inherit via internal rule
  Wplyw obrotow : DotProduct  OutDataTypeStr=Inherit: Inherit via internal rule
  Zaklocenia : Subsystem
  Zalaczony : DotProduct  OutDataTypeStr=Inherit: Inherit via internal rule
  "obr/min -> FS  " : Gain  Gain=1/1500
  "obr/min -> Hz" : Gain  Gain=1/60*2
  Obroty : Outport
  Prad : Outport  Port=2
  Idle : Outport  Port=3
  Running : Outport  Port=4
  Alarm : Outport  Port=5
  wires:
  Inercja mechaniczna/1 -> Obroty/1, Poslizg/1, Add1/2, "obr/min -> Hz"/1
  Sum/1 -> Inercja mechaniczna/1
  "Hz -> obr/min"/1 -> Sum2/1, Zaklocenia/1(In)  "[obr/min]"
  Poslizg/1 -> Sum/2
  Sum3/1 -> Poslizg/2
  Poslizg od obciazenia/1 -> Sum3/1
  Obciazenie zew/1 -> Saturation [0,1]/1  "FS"
  Poslizg jalowy/1 -> Sum3/2
  Prad nominalny (10A)/1 -> Prad jalowy/1  "A"
  Prad jalowy/1 -> Sum1/2, Wplyw obciazenia/2
  Wplyw obciazenia/1 -> Sum1/1
  Abs/1 -> Wplyw obciazenia/1  "FS"
  Const/1 -> Wplyw obrotow/1
  "obr/min -> Hz"/1 -> Sterownik/1(PV)
  Saturation [0,1]/1 -> Add/2
  Add/1 -> Poslizg od obciazenia/1, Abs/1  "FS"
  Add1/1 -> "obr/min -> FS  "/1
  "obr/min -> FS  "/1 -> Gain/1
  "Saturation [0,1] "/1 -> Add/1
  Zalaczenie/1 -> Sterowanie/2(Zalaczenie), Stan/1(Zalaczony)
  Sterowanie/1(Sterowanie) -> Sterownik/2(SP)
  Gain/1 -> "Saturation [0,1] "/1
  Uszkodzenie/1 -> Relay/1
  Sterownik/1(CV) -> Wplyw uszkodzenia/1
  Relay/1 -> Wplyw uszkodzenia/2, Stan/2(Zdatny)
  Wplyw uszkodzenia/1 -> "Hz -> obr/min"/1
  Wplyw obrotow/1 -> Prad/1  "A"
  Sum1/1 -> Zalaczony/1  "A"
  Zalaczony/1 -> Wplyw obrotow/2
  Zadane obroty/1 -> Sterowanie/1(Zadane obroty)
  Stan/1(Idle) -> Idle/1
  Stan/2(Running) -> Running/1, Zalaczony/2
  Stan/3(Alarm) -> Alarm/1
  Sum2/1 -> Add1/1, Sum/1
  Zaklocenia/1(Out) -> Sum2/2

== system BrowarModel/Mlyn browarniany/Mlyn browarniany/Walce mlyna/Komora nad walcami ==
  note: [0,1]
  note: Komora nad walcami
  Doplyw : Inport
  Odplyw : Inport  Port=2
  Detektory poziomu : Subsystem
  Integrator (max = 1m3) : Integrator  LimitOutput=on  UpperSaturationLimit=1  LowerSaturationLimit=0
  Sum : Sum  Inputs=|+-
  Wspolczynnik skalujacy : Gain  Gain=1/1
  Zmiana gestosci : Gain  Gain=1/0.9
  Stopien wypelnienie : Outport
  Poziom HI : Outport  Port=2
  Poziom LO : Outport  Port=3
  wires:
  Sum/1 -> Integrator (max = 1m3)/1  "m3/s"
  Integrator (max = 1m3)/1 -> Wspolczynnik skalujacy/1  "m3"
  Odplyw/1 -> Zmiana gestosci/1  "m3/s"
  Doplyw/1 -> Sum/1  "m3/s"
  Wspolczynnik skalujacy/1 -> Stopien wypelnienie/1, Detektory poziomu/1(Poziom)
  Zmiana gestosci/1 -> Sum/2
  Detektory poziomu/1(Poziom  wysoki) -> Poziom HI/1
  Detektory poziomu/2(Poziom niski) -> Poziom LO/1

== system BrowarModel/Mlyn browarniany/Mlyn browarniany/Walce mlyna/Silnik elektryczny ==
  note: Silnik elektryczny
  note: Uszkodzenie silnika
  Zalaczenie : Inport
  Zadane obroty : Inport  Port=2
  Obciazenie zew : Inport  Port=3
  Uszkodzenie : Inport  Port=4
  Abs : Abs  SaturateOnIntegerOverflow=off
  Add : Sum
  Add1 : Sum  Inputs=+-
  Const : Constant
  Gain : Gain
  "Hz -> obr/min" : Gain  Gain=60/2
  Inercja mechaniczna : TransferFcn  Denominator=[1 1]
  Poslizg : DotProduct  OutDataTypeStr=Inherit: Inherit via internal rule
  Poslizg jalowy : Constant  Value=0.04
  Poslizg od obciazenia : Gain  Gain=0.05
  Prad jalowy : Gain  Gain=0.5
  Prad nominalny (10A) : Constant  Value=10
  Relay : Relay  OnOutputValue=0  OffOutputValue=1
  Saturation [0,1] : Saturate  UpperLimit=1  LowerLimit=0
  "Saturation [0,1] " : Saturate  UpperLimit=1  LowerLimit=0
  Stan : Subsystem
  Sterowanie : Subsystem
  Sterownik : Subsystem
  Sum : Sum  Inputs=|+-
  Sum1 : Sum  Inputs=|++
  Sum2 : Sum  Inputs=|+-
  Sum3 : Sum  Inputs=|++
  Wplyw uszkodzenia : DotProduct  OutDataTypeStr=Inherit: Inherit via internal rule
  Wplyw obciazenia : DotProduct  OutDataTypeStr=Inherit: Inherit via internal rule
  Wplyw obrotow : DotProduct  OutDataTypeStr=Inherit: Inherit via internal rule
  Zaklocenia : Subsystem
  Zalaczony : DotProduct  OutDataTypeStr=Inherit: Inherit via internal rule
  "obr/min -> FS  " : Gain  Gain=1/1500
  "obr/min -> Hz" : Gain  Gain=1/60*2
  Obroty : Outport
  Prad : Outport  Port=2
  Idle : Outport  Port=3
  Running : Outport  Port=4
  Alarm : Outport  Port=5
  wires:
  Inercja mechaniczna/1 -> Obroty/1, Poslizg/1, Add1/2, "obr/min -> Hz"/1
  Sum/1 -> Inercja mechaniczna/1
  "Hz -> obr/min"/1 -> Sum2/1, Zaklocenia/1(In)  "[obr/min]"
  Poslizg/1 -> Sum/2
  Sum3/1 -> Poslizg/2
  Poslizg od obciazenia/1 -> Sum3/1
  Obciazenie zew/1 -> Saturation [0,1]/1  "FS"
  Poslizg jalowy/1 -> Sum3/2
  Prad nominalny (10A)/1 -> Prad jalowy/1  "A"
  Prad jalowy/1 -> Sum1/2, Wplyw obciazenia/2
  Wplyw obciazenia/1 -> Sum1/1
  Abs/1 -> Wplyw obciazenia/1  "FS"
  Const/1 -> Wplyw obrotow/1
  "obr/min -> Hz"/1 -> Sterownik/1(PV)
  Saturation [0,1]/1 -> Add/2
  Add/1 -> Poslizg od obciazenia/1, Abs/1  "FS"
  Add1/1 -> "obr/min -> FS  "/1
  "obr/min -> FS  "/1 -> Gain/1
  "Saturation [0,1] "/1 -> Add/1
  Zalaczenie/1 -> Sterowanie/2(Zalaczenie), Stan/1(Zalaczony)
  Sterowanie/1(Sterowanie) -> Sterownik/2(SP)
  Gain/1 -> "Saturation [0,1] "/1
  Uszkodzenie/1 -> Relay/1
  Sterownik/1(CV) -> Wplyw uszkodzenia/1
  Relay/1 -> Wplyw uszkodzenia/2, Stan/2(Zdatny)
  Wplyw uszkodzenia/1 -> "Hz -> obr/min"/1
  Wplyw obrotow/1 -> Prad/1  "A"
  Sum1/1 -> Zalaczony/1  "A"
  Zalaczony/1 -> Wplyw obrotow/2
  Zadane obroty/1 -> Sterowanie/1(Zadane obroty)
  Stan/1(Idle) -> Idle/1
  Stan/2(Running) -> Running/1, Zalaczony/2
  Stan/3(Alarm) -> Alarm/1
  Sum2/1 -> Add1/1, Sum/1
  Zaklocenia/1(Out) -> Sum2/2

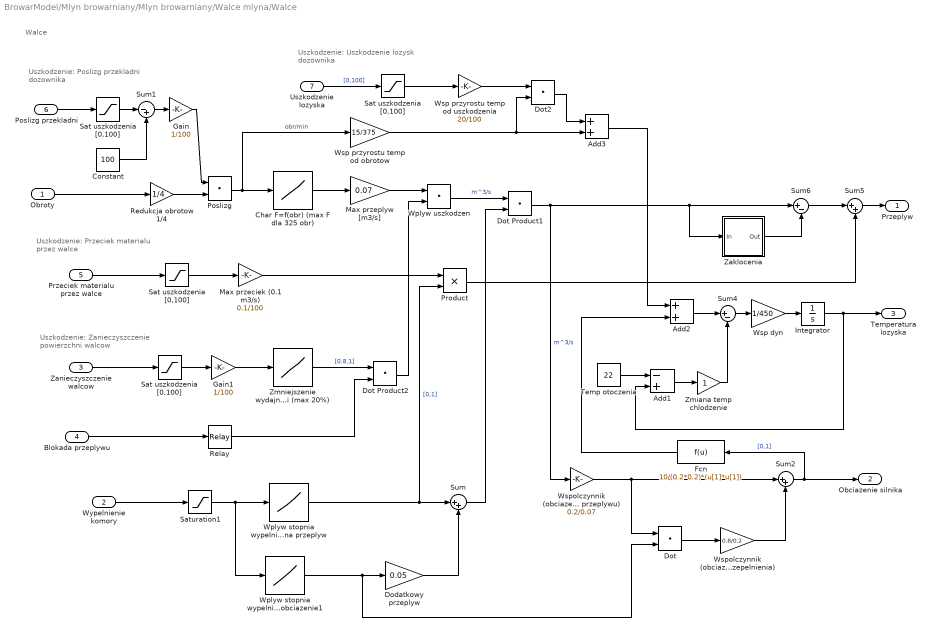
== system BrowarModel/Mlyn browarniany/Mlyn browarniany/Walce mlyna/Walce ==
  note: Uszkodzenie:
      | Poslizg przekladni dozownika
  note: Walce
  note: Uszkodzenie:
      | Uszkodzenie lozysk dozownika
  note: Uszkodzenie:
      | Zanieczyszczenie powierzchni walcow
  note: Uszkodzenie:
      | Przeciek materialu przez walce
  Obroty : Inport
  Wypelnienie komory : Inport  Port=2
  Zanieczyszczenie walcow : Inport  Port=3
  Blokada przeplywu : Inport  Port=4
  Przeciek materialu przez walce : Inport  Port=5
  Poslizg przekladni : Inport  Port=6
  Uszkodzenie lozyska : Inport  Port=7
  Add1 : Sum  Inputs=-+
  Add2 : Sum
  Add3 : Sum
  Char F=f(obr) (max F dla 325 obr) : Lookup  InputValues="[0\t25\t50\t75\t100\t125\t150\t175\t200\t225\t250\t275\t300\t325\t350\t375\t400\t425\t450]"  Table="[0.0000\t0.0777\t0.1550\t0.2315\t0.3067\t0.3803\t0.4519\t0.5209\t0.5871\t0.6500\t0.7092\t0.7643\t0.8148\t0.8604\t0.9007\t0.9352\t0.9635\t0.9853\t1.0000]"  SaturateOnIntegerOverflow=off
  Constant : Constant  Value=100
  Dodatkowy przeplyw : Gain  Gain=0.05
  Dot : DotProduct  OutDataTypeStr=Inherit: Inherit via internal rule
  Dot Product1 : DotProduct  OutDataTypeStr=Inherit: Inherit via internal rule
  Dot Product2 : DotProduct  OutDataTypeStr=Inherit: Inherit via internal rule
  Dot2 : DotProduct  OutDataTypeStr=Inherit: Inherit via internal rule
  Fcn : Fcn  Expr=10/(0.2*0.2)*(u[1]*u[1])
  Gain : Gain  Gain=1/100
  Gain1 : Gain  Gain=1/100
  Integrator : Integrator  InitialCondition=22  LimitOutput=on  LowerSaturationLimit=0
  Max przeciek (0.1 m3/s) : Gain  Gain=0.1/100
  Max przeplyw [m3/s] : Gain  Gain=0.07
  Poslizg : DotProduct  OutDataTypeStr=Inherit: Inherit via internal rule
  Product : Product  RndMeth=Zero
  Redukcja obrotow 1/4 : Gain  Gain=1/4
  Relay : Relay  OnOutputValue=0  OffOutputValue=1
  Sat uszkodzenia [0,100] : Saturate  UpperLimit=100  LowerLimit=0
  "Sat uszkodzenia [0,100] " : Saturate  UpperLimit=100  LowerLimit=0
  Sat uszkodzenia [0,100] : Saturate  UpperLimit=100  LowerLimit=0
  "Sat uszkodzenia [0,100] " : Saturate  UpperLimit=100  LowerLimit=0
  Saturation1 : Saturate  UpperLimit=1  LowerLimit=0
  Sum : Sum  Inputs=|++
  Sum1 : Sum  Inputs=|-+
  Sum2 : Sum  Inputs=|++
  Sum4 : Sum  Inputs=|+-
  Sum5 : Sum  Inputs=|++
  Sum6 : Sum  Inputs=|+-
  Temp otoczenia : Constant  Value=22
  Wplyw uszkodzen : DotProduct  OutDataTypeStr=Inherit: Inherit via internal rule
  Wplyw stopnia wypelnienia na przeplyw : Lookup  InputValues=[-1,0,0.1,1]  Table=[0,0,1,1]  SaturateOnIntegerOverflow=off
  Wplyw stopnia wypelnienia na przeplyw i obciazenie1 : Lookup  InputValues=[0,0.9,1,2]  Table=[0,0,1,1]  SaturateOnIntegerOverflow=off
  Wsp dyn : Gain  Gain=1/450
  Wsp przyrostu temp od obrotow : Gain  Gain=15/375
  Wsp przyrostu temp od uszkodzenia : Gain  Gain=20/100
  Wspolczynnik (obciazenie od przepelnienia) : Gain  Gain=0.8/0.2
  Wspolczynnik (obciazenie od przeplywu) : Gain  Gain=0.2/0.07
  Zaklocenia : Subsystem
  Zmiana temp chlodzenie : Gain
  Zmniejszenie wydajnosci (max 20%) : Lookup  InputValues=[-1, 0, 1, 2]  Table=[1, 1, 0.8, 0.8]  SaturateOnIntegerOverflow=off
  Przeplyw : Outport
  Obciazenie silnika : Outport  Port=2
  Temperatura lozyska : Outport  Port=3
  wires:
  Char F=f(obr) (max F dla 325 obr)/1 -> Max przeplyw [m3/s]/1
  Max przeplyw [m3/s]/1 -> Wplyw uszkodzen/1
  Zanieczyszczenie walcow/1 -> Sat uszkodzenia [0,100]/1
  Poslizg/1 -> Char F=f(obr) (max F dla 325 obr)/1, Wsp przyrostu temp od obrotow/1  "obr/min"
  Poslizg przekladni/1 -> Sat uszkodzenia [0,100]/1
  Sat uszkodzenia [0,100]/1 -> Sum1/1
  Sum1/1 -> Gain/1
  Constant/1 -> Sum1/2
  Obroty/1 -> Redukcja obrotow 1/4/1
  Redukcja obrotow 1/4/1 -> Poslizg/2
  Sat uszkodzenia [0,100]/1 -> Gain1/1
  Wypelnienie komory/1 -> Saturation1/1
  Saturation1/1 -> Wplyw stopnia wypelnienia na przeplyw/1, Wplyw stopnia wypelnienia na przeplyw i obciazenie1/1
  Wplyw uszkodzen/1 -> Dot Product1/1  "m^3/s"
  Dot Product1/1 -> Wspolczynnik (obciazenie od przeplywu)/1, Sum6/1, Zaklocenia/1(In)  "m^3/s"
  Wplyw stopnia wypelnienia na przeplyw i obciazenie1/1 -> Dodatkowy przeplyw/1, Dot/2
  Sum/1 -> Dot Product1/2
  Wplyw stopnia wypelnienia na przeplyw/1 -> Sum/1, Product/2  "[0,1]"
  Dodatkowy przeplyw/1 -> Sum/2
  Sum2/1 -> Fcn/1, Obciazenie silnika/1  "[0,1]"
  Dot/1 -> Wspolczynnik (obciazenie od przepelnienia)/1
  Wspolczynnik (obciazenie od przepelnienia)/1 -> Sum2/2
  Wspolczynnik (obciazenie od przeplywu)/1 -> Dot/1, Sum2/1
  Uszkodzenie lozyska/1 -> "Sat uszkodzenia [0,100] "/1  "[0,100]"
  "Sat uszkodzenia [0,100] "/1 -> Wsp przyrostu temp od uszkodzenia/1
  Wsp przyrostu temp od uszkodzenia/1 -> Dot2/1
  Sum4/1 -> Wsp dyn/1
  Integrator/1 -> Add1/2, Temperatura lozyska/1
  Add1/1 -> Zmiana temp chlodzenie/1
  Zmiana temp chlodzenie/1 -> Sum4/2
  Add2/1 -> Sum4/1
  Temp otoczenia/1 -> Add1/1
  Blokada przeplywu/1 -> Relay/1
  Zmniejszenie wydajnosci (max 20%)/1 -> Dot Product2/1  "[0.8,1]"
  Relay/1 -> Dot Product2/2
  Dot Product2/1 -> Wplyw uszkodzen/2
  Wsp przyrostu temp od obrotow/1 -> Dot2/2, Add3/2
  Dot2/1 -> Add3/1
  Add3/1 -> Add2/1
  Fcn/1 -> Add2/2
  Wsp dyn/1 -> Integrator/1
  Sum5/1 -> Przeplyw/1
  Sum6/1 -> Sum5/1
  Zaklocenia/1(Out) -> Sum6/2
  Gain/1 -> Poslizg/1
  Gain1/1 -> Zmniejszenie wydajnosci (max 20%)/1
  "Sat uszkodzenia [0,100] "/1 -> Max przeciek (0.1 m3/s)/1
  Max przeciek (0.1 m3/s)/1 -> Product/1
  Przeciek materialu przez walce/1 -> "Sat uszkodzenia [0,100] "/1
  Product/1 -> Sum5/2
